simulink model "electricalfaults"  (R2023a)
settings: Solver=VariableStepAuto  StartTime=0.0  StopTime=10.0  RelTol=1e-3
libraries: spsVoltageMeasurementLib x4, spsACVoltageSourceLib x3, spsAsynchronousMachinepuUnitsLib x1, spsGroundLib x1, spsTHDLib x1, spspowerguiLib x1
settings Model: Creator=admin  LastModifiedBy=admin

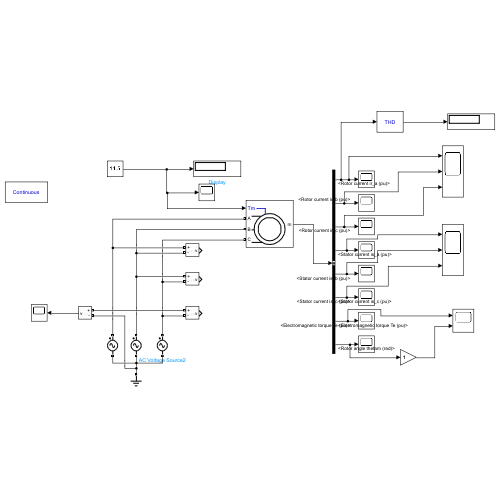
[thumbnail: Simulink's stored preview of the top-level diagram]
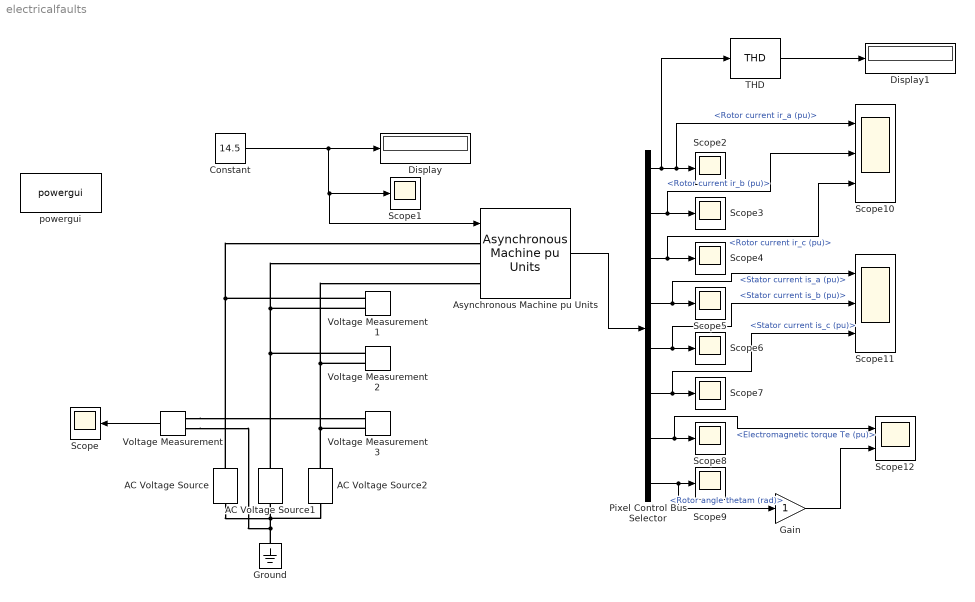
== system electricalfaults ==
  AC Voltage Source : spsACVoltageSourceLib/AC Voltage Source  Amplitude=100  Phase=0  Frequency=60  SampleTime=0  Measurements=None  BusType=swing  Pref=10e3  Qref=0  Qmin=-inf  Qmax=+inf
  AC Voltage Source1 : spsACVoltageSourceLib/AC Voltage Source  Amplitude=100  Phase=0  Frequency=60  SampleTime=0  Measurements=None  BusType=swing  Pref=10e3  Qref=0  Qmin=-inf  Qmax=+inf
  AC Voltage Source2 : spsACVoltageSourceLib/AC Voltage Source  Amplitude=100  Phase=0  Frequency=60  SampleTime=0  Measurements=None  BusType=swing  Pref=10e3  Qref=0  Qmin=-inf  Qmax=+inf
  Asynchronous Machine pu Units : spsAsynchronousMachinepuUnitsLib/Asynchronous Machine pu Units  RotorType=Squirrel-cage  PresetModel=No  MechanicalLoad=Torque Tm  ShowDetailedParameters=on  ReferenceFrame=Rotor  Units=pu  MeasurementBus=off  NominalParameters=[3730 460 60]  VoltageRatio=1  Stator=[0.01965 0.0397]  Rotor=[0.01909 0.0397]  Cage1=[0.01909 0.0397]  Cage2=[0.01909 0.0397]  Lm=1.354  Mechanical=[0.09526 0.05479 2]  PolePairs=2  InitialConditions="[ 1,0   0,0,0   0,0,0 ]"  SimulateSaturation=off  Saturation="[0.212,0.4201,0.8125,1.0979,1.4799,2.2457,3.2586,4.5763,6.4763 ;   0.5,0.7,0.9,1,1.1,1.2 ,1.3,1.4,1.5]"  LoadFlowParameters=0  TsPowergui=0  TsBlock=-1  IterativeModel=Trapezoidal non iterative  IterativeDiscreteModel=Trapezoidal non iterative  Pmec=0
      settings: LibrarySourceBlock=|
      | sps_lib/Electrical Machines/Asynchronous Machine
      | pu Units
  Constant : Constant  Value=14.5
  Display : Display
  Display1 : Display
  Gain : Gain
  Ground : spsGroundLib/Ground  LConnTagsString=a
  Pixel Control Bus Selector : BusSelector  OutputSignals=Rotor measurements.Rotor current ir_a (pu),Rotor measurements.Rotor current ir_b (pu),Rotor measurements.Rotor current ir_c (pu),Stator measurements.Stator current is_a (pu),Stator measurements.Stator current is_b (pu),Stator measurements.Stator current is_c (pu),Mechanical.Electromagnetic torque Te (pu),Mechanical.Rotor angle thetam (rad)
  Scope{,1..9} (10 alike) : Scope
  Scope10 : Scope  NumInputPorts=3
  Scope11 : Scope  NumInputPorts=3
  Scope12 : Scope  NumInputPorts=2
  THD : spsTHDLib/THD  Freq=60  Ts=0
  Voltage Measurement{,1..3} (4 alike) : spsVoltageMeasurementLib/Voltage Measurement  PhasorSimulation=off  OutputType=Complex  PSBequivalent=0
  powergui : spspowerguiLib/powergui  Priority=1  SimulationMode=Continuous  SampleTime=50e-6  frequency=60  Iterations=50  frequencyindice=60  Pbase=100e6  ErrMax=1e-4  UnitsV=kV  UnitsW=MW  buscounter=0  FunctionMessages=off  echomessages=off  EnableUseOfTLC=off  CurrentSourceSwitches=off  DisableSnubberDevices=off  DisableRonSwitches=off  DisableVfSwitches=off  DisplayEquations=off  AutomaticDiscreteSolvers=off  SolverType=Tustin/Backward Euler (TBE)  Interpol=off  ExternalGateDelay=off  methode=off  Ts=100  x0status=blocks  SPID=on  SwTol=0  HookPort=off  NonlinearTolerance=1e-4  nMaxIteration=100  ContinueOnMaxIteration=off  RestoreLinks=warning  ResistiveCurrentMeasurement=off  Frange=[0:2:500]  Ylog=off  Xlog=on  ShowGrid=off  save=off  variable=ZData  structure=0  ZoomFFT=off  StartTime=0.0  cycles=1  DisplayStyle=1  fundamental=60  FreqAxis=off  MaxFrequency=1000  frequencyindicesteady=1  RmsSteady=1  display=off
  wires:
  Voltage Measurement/1 -> Scope/1
  Constant/1 -> Asynchronous Machine pu Units/1, Scope1/1, Display/1
  Asynchronous Machine pu Units/1 -> Pixel Control Bus Selector/1
  Pixel Control Bus Selector/1 -> THD/1, Scope10/1, Scope2/1  "<Rotor current ir_a (pu)>"
  Pixel Control Bus Selector/2 -> Scope10/2, Scope3/1  "<Rotor current ir_b (pu)>"
  Pixel Control Bus Selector/3 -> Scope10/3, Scope4/1  "<Rotor current ir_c (pu)>"
  Pixel Control Bus Selector/4 -> Scope11/1, Scope5/1  "<Stator current is_a (pu)>"
  Pixel Control Bus Selector/5 -> Scope11/2, Scope6/1  "<Stator current is_b (pu)>"
  Pixel Control Bus Selector/6 -> Scope11/3, Scope7/1  "<Stator current is_c (pu)>"
  Pixel Control Bus Selector/7 -> Scope12/1, Scope8/1  "<Electromagnetic torque Te (pu)>"
  Pixel Control Bus Selector/8 -> Gain/1, Scope9/1  "<Rotor angle thetam (rad)>"
  Gain/1 -> Scope12/2
  THD/1 -> Display1/1
  connections:
  Voltage Measurement/LConn1 -- Voltage Measurement3/LConn1
  AC Voltage Source/RConn1 -- Voltage Measurement1/LConn1 -- Asynchronous Machine pu Units/LConn1
  AC Voltage Source1/RConn1 -- Voltage Measurement2/LConn1 -- Voltage Measurement1/LConn2 -- Asynchronous Machine pu Units/LConn2
  AC Voltage Source2/RConn1 -- Voltage Measurement3/LConn2 -- Voltage Measurement2/LConn2 -- Asynchronous Machine pu Units/LConn3
  Ground/LConn1 -- Voltage Measurement/LConn2 -- AC Voltage Source2/LConn1 -- AC Voltage Source/LConn1 -- AC Voltage Source1/LConn1
